simulink model "sim_dwupunktowy_pogodowa"  (R2023b)
settings: Solver=VariableStepAuto  StartTime=0.0  StopTime=10.0  MaxStep=0.01  RelTol=1e-3
undefined symbols (not defined in the file): k, ki, kp, T, T_oz0, To
settings Model: Creator=tomasz  LastModifiedBy=tomasz

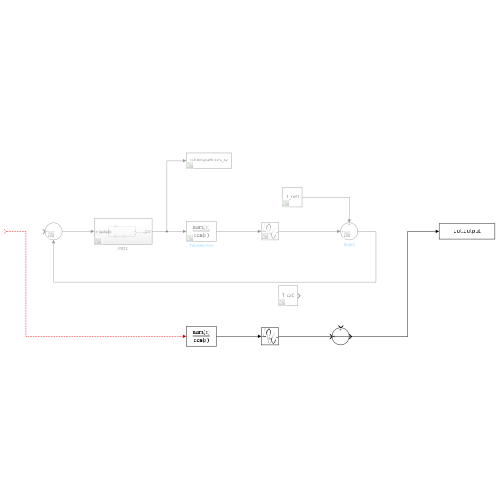
[thumbnail: Simulink's stored preview of the top-level diagram]
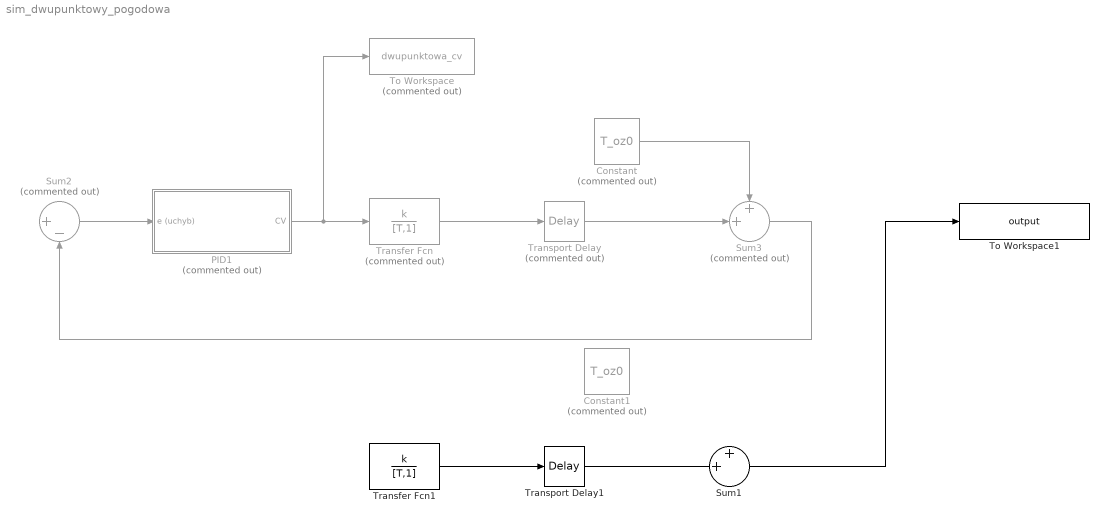
== system sim_dwupunktowy_pogodowa ==
  Constant : Constant  Commented=on  Value=T_oz0
  Constant1 : Constant  Commented=on  Value=T_oz0
  PID1 : Subsystem  Commented=on
  Sum1 : Sum  Inputs=++|
  Sum2 : Sum  Commented=on  Inputs=|+-
  Sum3 : Sum  Commented=on  Inputs=++|
  To Workspace : ToWorkspace  Commented=on  VariableName=dwupunktowa_cv  SampleTime=-1
  To Workspace1 : ToWorkspace  VariableName=output  SampleTime=-1
  Transfer Fcn : TransferFcn  Commented=on  Numerator=k  Denominator=[T,1]
  Transfer Fcn1 : TransferFcn  Numerator=k  Denominator=[T,1]
  Transport Delay : TransportDelay  Commented=on  DelayTime=To
  Transport Delay1 : TransportDelay  DelayTime=To
  wires:
  Sum2/1 -> PID1/1(e (uchyb))
  PID1/1(CV) -> To Workspace/1, Transfer Fcn/1
  Sum3/1 -> Sum2/2
  Constant/1 -> Sum3/1
  Transfer Fcn/1 -> Transport Delay/1
  Transport Delay/1 -> Sum3/2
  Transfer Fcn1/1 -> Transport Delay1/1
  Transport Delay1/1 -> To Workspace1/1
  ? -> Transfer Fcn1/1

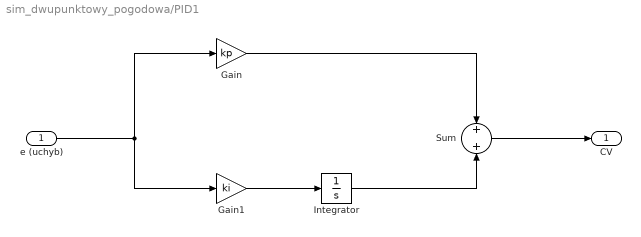
== system sim_dwupunktowy_pogodowa/PID1 ==
  e (uchyb) : Inport
  Gain : Gain  Gain=kp
  Gain1 : Gain  Gain=ki
  Integrator : Integrator
  Sum : Sum
  CV : Outport
  wires:
  Integrator/1 -> Sum/2
  Gain1/1 -> Integrator/1
  Gain/1 -> Sum/1
  e (uchyb)/1 -> Gain1/1, Gain/1
  Sum/1 -> CV/1
